simulink model "wahWahEffect"  (R2022b)
settings: Solver=FixedStepDiscrete  StartTime=0.0  StopTime=simParams.stopTime  RelTol=1e-3
PostLoadFcn:
  | postLoadCallback
InitFcn:
  | initCallback
StopFcn:
  | stopCallback
undefined symbols (not defined in the file or in its folder): modelParams
libraries: dspsrcs4 x8, hdlsllib x1
CloseFcn:
  | closeCallback
settings Model: DataTypeOverride=Off  PacingRate=0.110000  Creator=foruf  LastModifiedBy=Sohai
settings DataIOCC: ReturnWorkspaceOutputs=off
settings OptimizationCC: BlockReduction=off  ConditionallyExecuteInputs=off  DefaultParameterBehavior=Inlined  InheritOutputTypeSmallerThanSingle=on
settings DebuggingCC: AlgebraicLoopMsg=error  SingleTaskRateTransMsg=error
settings HardwareCC: ProdBitPerPointer=32  ProdBitPerSizeT=32  ProdBitPerPtrDiffT=32  ProdLargestAtomicFloat=None  ProdIntDivRoundTo=Undefined  ProdEndianess=Unspecified  ProdWordSize=32  ProdHWDeviceType=ASIC/FPGA->ASIC/FPGA  TargetBitPerPointer=64  TargetBitPerSizeT=64  TargetBitPerPtrDiffT=64  TargetLongLongMode=on  TargetIntDivRoundTo=Zero  TargetEndianess=LittleEndian  TargetWordSize=64  TargetHWDeviceType=Custom Processor->MATLAB Host Computer  ProdEqTarget=off
settings ModelReferenceCC: EnableRefExpFcnMdlSchedulingChecks=on

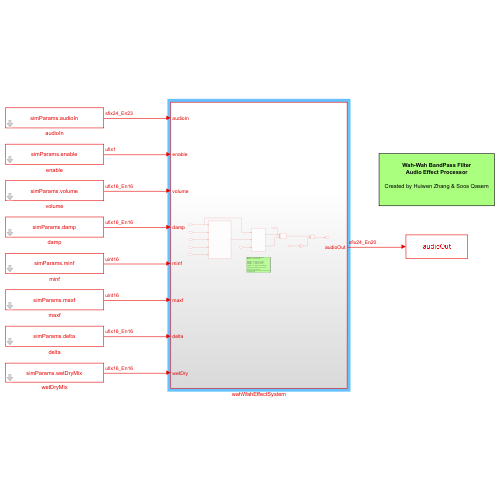
[thumbnail: Simulink's stored preview of the top-level diagram]
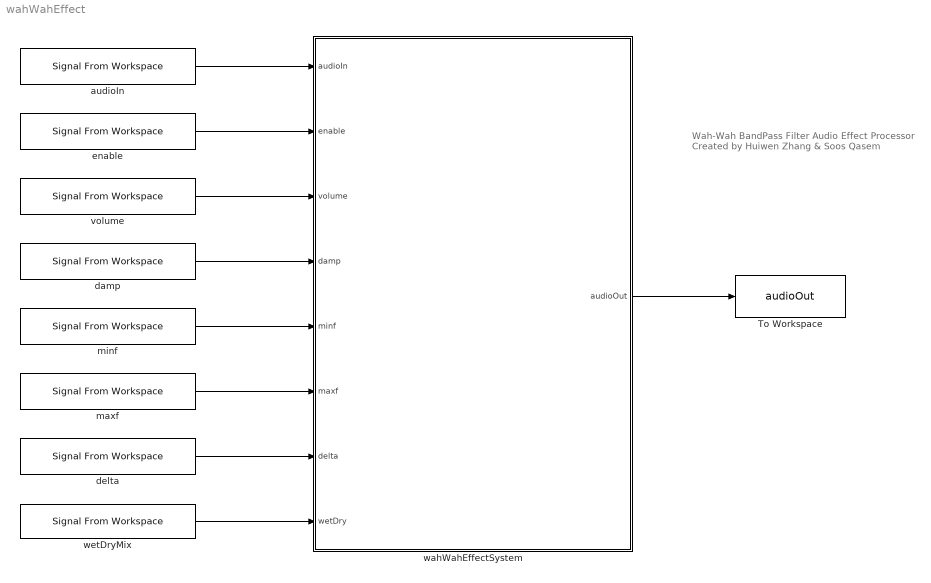
== system wahWahEffect ==
  note: Wah-Wah BandPass Filter
      | Audio Effect Processor
      |
      | Created by Huiwen Zhang & Soos Qasem
  To Workspace : ToWorkspace  VariableName=audioOut  SampleTime=-1
      settings: Save2DSignal=2-D array (concatenate along first dimension)
  audioIn : dspsrcs4/Signal From Workspace  X=simParams.audioIn  Ts=modelParams.audio.samplePeriod  nsamps=1  OutputAfterFinalValue=Setting to zero  ignoreOrWarnInputAndFrameLengths=off  OutputFrames=off
  damp : dspsrcs4/Signal From Workspace  X=simParams.damp  Ts=modelParams.audio.samplePeriod  nsamps=1  OutputAfterFinalValue=Holding final value  ignoreOrWarnInputAndFrameLengths=off  OutputFrames=off
  delta : dspsrcs4/Signal From Workspace  X=simParams.delta  Ts=modelParams.audio.samplePeriod  nsamps=1  OutputAfterFinalValue=Holding final value  ignoreOrWarnInputAndFrameLengths=off  OutputFrames=off
  enable : dspsrcs4/Signal From Workspace  X=simParams.enable  Ts=modelParams.audio.samplePeriod  nsamps=1  OutputAfterFinalValue=Holding final value  ignoreOrWarnInputAndFrameLengths=off  OutputFrames=off
  maxf : dspsrcs4/Signal From Workspace  X=simParams.maxf  Ts=modelParams.audio.samplePeriod  nsamps=1  OutputAfterFinalValue=Holding final value  ignoreOrWarnInputAndFrameLengths=off  OutputFrames=off
  minf : dspsrcs4/Signal From Workspace  X=simParams.minf  Ts=modelParams.audio.samplePeriod  nsamps=1  OutputAfterFinalValue=Holding final value  ignoreOrWarnInputAndFrameLengths=off  OutputFrames=off
  volume : dspsrcs4/Signal From Workspace  X=simParams.volume  Ts=modelParams.audio.samplePeriod  nsamps=1  OutputAfterFinalValue=Holding final value  ignoreOrWarnInputAndFrameLengths=off  OutputFrames=off
  wahWahEffectSystem : Subsystem
  wetDryMix : dspsrcs4/Signal From Workspace  X=simParams.wetDryMix  Ts=modelParams.audio.samplePeriod  nsamps=1  OutputAfterFinalValue=Holding final value  ignoreOrWarnInputAndFrameLengths=off  OutputFrames=off
  wires:
  audioIn/1 -> wahWahEffectSystem/1(audioIn)
  enable/1 -> wahWahEffectSystem/2(enable)
  volume/1 -> wahWahEffectSystem/3(volume)
  damp/1 -> wahWahEffectSystem/4(damp)
  wahWahEffectSystem/1(audioOut) -> To Workspace/1
  minf/1 -> wahWahEffectSystem/5(minf)
  maxf/1 -> wahWahEffectSystem/6(maxf)
  delta/1 -> wahWahEffectSystem/7(delta)
  wetDryMix/1 -> wahWahEffectSystem/8(wetDry)

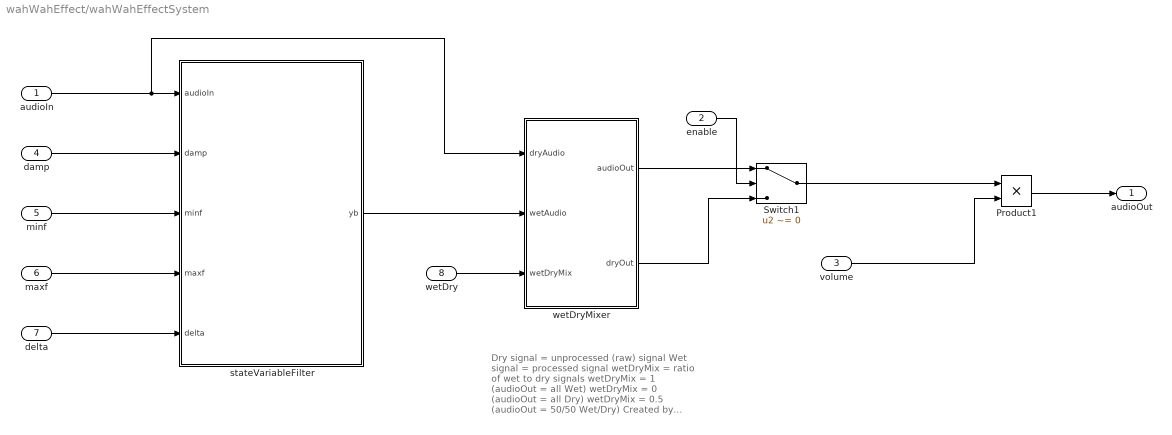
== system wahWahEffect/wahWahEffectSystem ==
  note: Dry signal = unprocessed (raw) signal
      | Wet signal = processed signal
      |
      | wetDryMix = ratio of wet to dry signals
      | wetDryMix = 1 (audioOut = all Wet)
      | wetDryMix = 0 (audioOut = all Dry)
      | wetDryMix = 0.5 (audioOut = 50/50 Wet/Dry)
      |
      | Created by Ross Snider and Trevor Vannoy
      | SPDX-License-Identifier: MIT
      | Copyright (c) 2022 Ross K. Snider & Trevor Vannoy
      | All rights reserved.
  audioIn : Inport
  enable : Inport  Port=2
  volume : Inport  Port=3  OutMin=[0]
  damp : Inport  Port=4  OutMin=[0]
  minf : Inport  Port=5  OutMin=[0]
  maxf : Inport  Port=6  OutMin=[0]
  delta : Inport  Port=7  OutMin=[0]
  wetDry : Inport  Port=8
  Product1 : Product  OutDataTypeStr=fixdt(1,24,20)
  Switch1 : Switch  Criteria=u2 ~= 0  Threshold=1  SaturateOnIntegerOverflow=off  InputSameDT=off
  stateVariableFilter : Subsystem
  wetDryMixer : Subsystem
  audioOut : Outport
  wires:
  audioIn/1 -> wetDryMixer/1(dryAudio), stateVariableFilter/1(audioIn)
  damp/1 -> stateVariableFilter/2(damp)
  enable/1 -> Switch1/2
  wetDryMixer/2(dryOut) -> Switch1/3
  volume/1 -> Product1/2
  wetDryMixer/1(audioOut) -> Switch1/1
  wetDry/1 -> wetDryMixer/3(wetDryMix)
  maxf/1 -> stateVariableFilter/4(maxf)
  minf/1 -> stateVariableFilter/3(minf)
  Switch1/1 -> Product1/1
  delta/1 -> stateVariableFilter/5(delta)
  Product1/1 -> audioOut/1
  stateVariableFilter/1(yb) -> wetDryMixer/2(wetAudio)

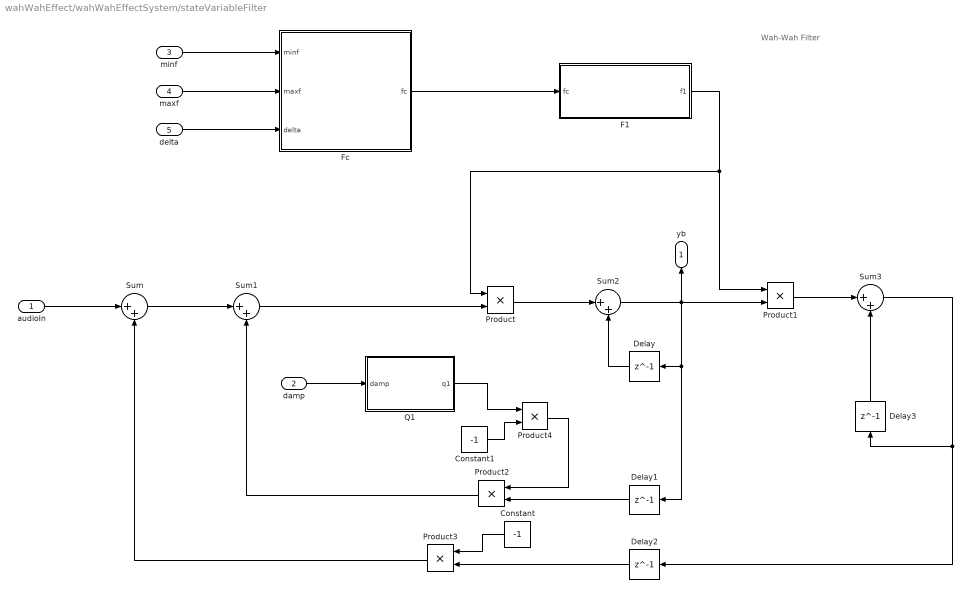
== system wahWahEffect/wahWahEffectSystem/stateVariableFilter ==
  note: Wah-Wah Filter
  audioIn : Inport
  damp : Inport  Port=2
  minf : Inport  Port=3
  maxf : Inport  Port=4
  delta : Inport  Port=5
  Constant : Constant  Value=-1  OutDataTypeStr=fixdt(1,2,0)  SampleTime=modelParams.audio.samplePeriod
  Constant1 : Constant  Value=-1  OutDataTypeStr=fixdt(1,2,0)  SampleTime=modelParams.audio.samplePeriod
  Delay{,1..3} (4 alike) : Delay  DelayLength=1  InitialCondition=0
  F1 : Subsystem
  Fc : Subsystem
  Product{,1..2,4} (4 alike) : Product  OutDataTypeStr=fixdt(1,24,23)
  Product3 : Product  OutDataTypeStr=fixdt(1,24,20)
  Q1 : Subsystem
  Sum{,1..3} (4 alike) : Sum  Inputs=|++  OutDataTypeStr=fixdt(1,24,20)  SaturateOnIntegerOverflow=on
  yb : Outport
  wires:
  audioIn/1 -> Sum/1
  Product1/1 -> Sum3/1
  Sum3/1 -> Delay3/1, Delay2/1
  Delay1/1 -> Product2/2
  Product2/1 -> Sum1/2
  Sum1/1 -> Product/2
  Constant/1 -> Product3/1
  Delay2/1 -> Product3/2
  Product3/1 -> Sum/2
  Product/1 -> Sum2/1
  Sum2/1 -> Delay1/1, Delay/1, yb/1, Product1/2
  Delay/1 -> Sum2/2
  minf/1 -> Fc/1(minf)
  maxf/1 -> Fc/2(maxf)
  delta/1 -> Fc/3(delta)
  Constant1/1 -> Product4/2
  Sum/1 -> Sum1/1
  Product4/1 -> Product2/1
  damp/1 -> Q1/1(damp)
  Q1/1(q1) -> Product4/1
  Fc/1(fc) -> F1/1(fc)
  F1/1(f1) -> Product1/1, Product/1
  Delay3/1 -> Sum3/2

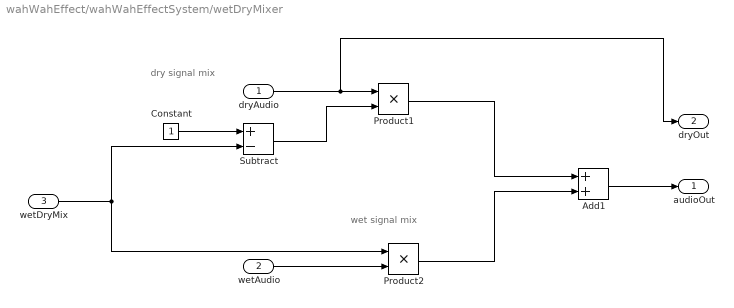
== system wahWahEffect/wahWahEffectSystem/wetDryMixer ==
  note: wet signal mix
  note: dry signal mix
  dryAudio : Inport
  wetAudio : Inport  Port=2
  wetDryMix : Inport  Port=3
  Add1 : Sum  OutDataTypeStr=fixdt(1,24,20)  SaturateOnIntegerOverflow=on
  Constant : Constant  OutDataTypeStr=fixdt(0,1,0)  SampleTime=modelParams.audio.samplePeriod
  Product1 : Product  OutDataTypeStr=fixdt(1,24,23)
  Product2 : Product  OutDataTypeStr=fixdt(1,24,20)
  Subtract : Sum  Inputs=+-  SaturateOnIntegerOverflow=on
  audioOut : Outport
  dryOut : Outport  Port=2
  wires:
  Product2/1 -> Add1/2
  Add1/1 -> audioOut/1
  Product1/1 -> Add1/1
  Constant/1 -> Subtract/1
  wetAudio/1 -> Product2/2
  Subtract/1 -> Product1/2
  wetDryMix/1 -> Product2/1, Subtract/2
  dryAudio/1 -> dryOut/1, Product1/1

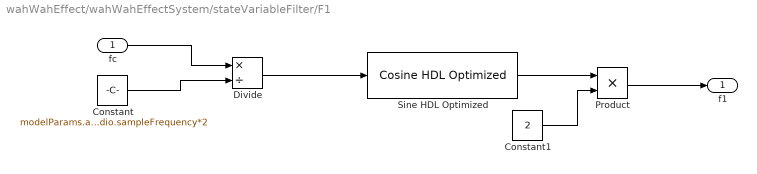
== system wahWahEffect/wahWahEffectSystem/stateVariableFilter/F1 ==
  fc : Inport
  Constant : Constant  Value=modelParams.audio.sampleFrequency*2  OutDataTypeStr=fixdt(1,32,0)  SampleTime=modelParams.audio.samplePeriod
  Constant1 : Constant  Value=2  OutDataTypeStr=fixdt(0,2,0)  SampleTime=modelParams.audio.samplePeriod
  Divide : Product  Inputs=*/  RndMeth=Zero  SaturateOnIntegerOverflow=on
  Product : Product  OutDataTypeStr=fixdt(1,24,23)
  Sine HDL Optimized : hdlsllib/Lookup Tables/Cosine HDL Optimized  OutputFormula=sin(2*pi*u)  NumDataPoints=1024  TableDataTypeStr=fixdt(1,31,31)  SimulateLUTROMDelay=off
      settings: LibrarySourceBlock=|
      | hdlsllib/Lookup
      | Tables/Sine
      | HDL Optimized
  f1 : Outport
  wires:
  fc/1 -> Divide/1
  Constant/1 -> Divide/2
  Sine HDL Optimized/1 -> Product/1
  Divide/1 -> Sine HDL Optimized/1
  Constant1/1 -> Product/2
  Product/1 -> f1/1

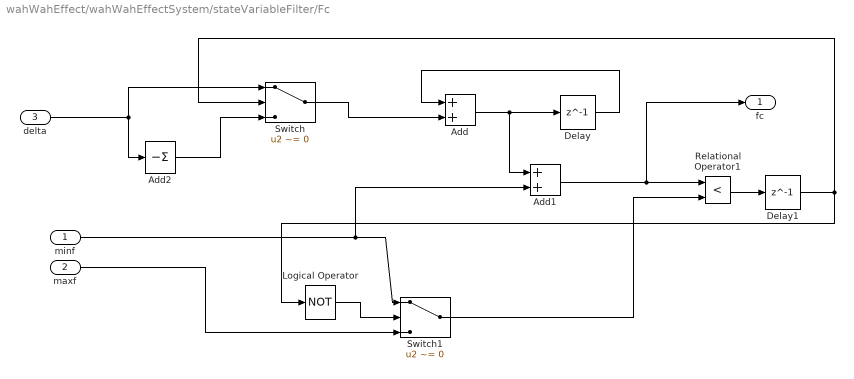
== system wahWahEffect/wahWahEffectSystem/stateVariableFilter/Fc ==
  minf : Inport
  maxf : Inport  Port=2
  delta : Inport  Port=3
  Add : Sum  OutDataTypeStr=fixdt(1,34,16)  SaturateOnIntegerOverflow=on
  Add1 : Sum  OutDataTypeStr=fixdt(1,34,16)  SaturateOnIntegerOverflow=on
  Add2 : Sum  Inputs=-
  Delay : Delay  DelayLength=1  InitialCondition=0
  Delay1 : Delay  DelayLength=1  InitialCondition=0
  Logical Operator : Logic  Operator=NOT  AllPortsSameDT=off  OutDataTypeStr=boolean
  Relational Operator1 : RelationalOperator  Operator=<  OutDataTypeStr=boolean  InputSameDT=off
  Switch : Switch  Criteria=u2 ~= 0  SaturateOnIntegerOverflow=off  InputSameDT=off
  Switch1 : Switch  Criteria=u2 ~= 0  SaturateOnIntegerOverflow=off  InputSameDT=off
  fc : Outport
  wires:
  Add/1 -> Delay/1, Add1/1
  Logical Operator/1 -> Switch1/2
  maxf/1 -> Switch1/3
  Add2/1 -> Switch/3
  minf/1 -> Add1/2, Switch1/1
  Switch/1 -> Add/2
  Switch1/1 -> Relational Operator1/2
  Delay/1 -> Add/1
  Relational Operator1/1 -> Delay1/1
  Delay1/1 -> Logical Operator/1, Switch/2
  delta/1 -> Add2/1, Switch/1
  Add1/1 -> fc/1, Relational Operator1/1

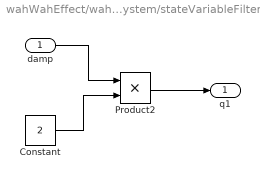
== system wahWahEffect/wahWahEffectSystem/stateVariableFilter/Q1 ==
  damp : Inport
  Constant : Constant  Value=2  OutDataTypeStr=fixdt(0,2,0)  SampleTime=modelParams.audio.samplePeriod
  Product2 : Product  OutDataTypeStr=fixdt(1,24,23)
  q1 : Outport
  wires:
  damp/1 -> Product2/1
  Constant/1 -> Product2/2
  Product2/1 -> q1/1
